simulink model "a"  (R2015a)
settings: Solver=ode3  StartTime=0.0  StopTime=20  FixedStep=2e-5  RelTol=2e-5
libraries: commchan3 x1, dsparch4 x1, commsink2 x1, commutil2 x1, commrandsrc2 x1, dspsigops x1
settings Model: Creator=Win 10  LastModifiedBy=Win 10

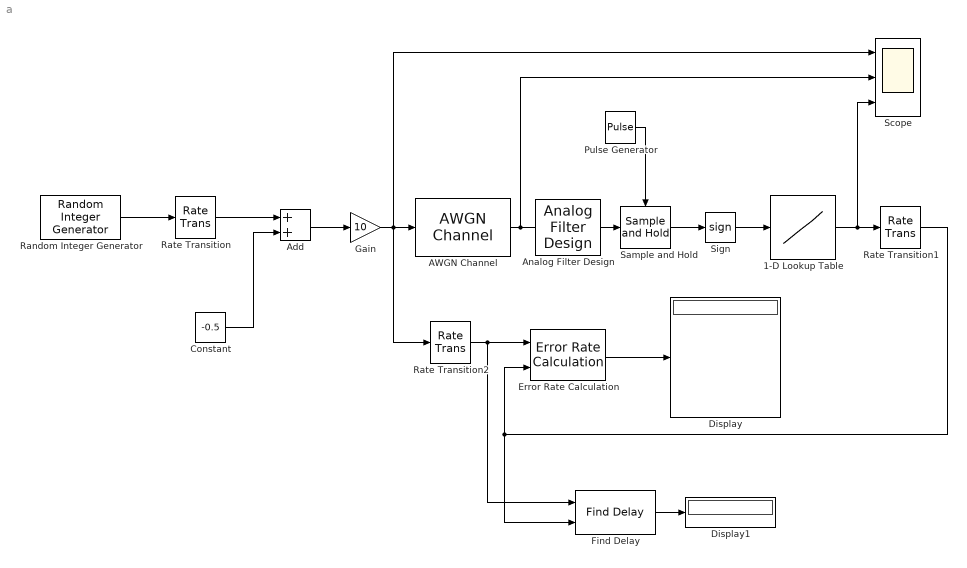
== system a ==
  1-D Lookup Table : Lookup_n-D  NumberOfTableDimensions=1  BreakpointsForDimension1=[-5:5]  Table=tanh([-5:5])  InternalRulePriority=Speed  RndMeth=Simplest  InputSameDT=on
  AWGN Channel : commchan3/AWGN Channel  InputProcessing=Columns as channels (frame based)  seed=67  noiseMode=Variance from mask  EbNodB=10  EsNodB=10  SNRdB=10  bitsPerSym=1  Ps=1  Tsym=1  variance=0
  Add : Sum
  Analog Filter Design : dsparch4/Analog Filter Design  method=Chebyshev I  filttype=Lowpass  N=9  Wlo=1200  Whi=80  Rp=0.1  Rs=40
  Constant : Constant  Value=-0.5
  Display : Display
      settings: Decimation=3
  Display1 : Display
  Error Rate Calculation : commsink2/Error Rate Calculation  N=0  st_delay=0  cp_mode=Entire frame  subframe=[]  PMode=Port  WsName=ErrorVec  RsMode2=off  stop=off  numErr=100  maxBits=1e6
  Find Delay : commutil2/Find Delay  corrLength=200  chgSigOP=off  stopUpdate=off  numConstDelay=3
  Gain : Gain  Gain=10
  Pulse Generator : DiscretePulseGenerator  PulseType=Time based  Period=1/2000  PulseWidth=20
  Random Integer Generator : commrandsrc2/Random Integer Generator  mul=2  seed=37  Ts=1/1000  frameBased=off  sampPerFrame=1  orient=off  outDataType=double
  Rate Transition : RateTransition
  Rate Transition1 : RateTransition  OutPortSampleTime=1/1000
  Rate Transition2 : RateTransition  OutPortSampleTime=1/1000
  Sample and Hold : dspsigops/Sample and Hold  trig=Rising edge  initCond=0  latchinput=off
  Scope : Scope  NumInputPorts=3
      settings: YMin=-5~-5~-5  YMax=5~5~5
  Sign : Signum
  wires:
  Random Integer Generator/1 -> Rate Transition/1
  Rate Transition/1 -> Add/1
  Constant/1 -> Add/2
  Add/1 -> Gain/1
  Gain/1 -> Rate Transition2/1, Scope/1, AWGN Channel/1
  AWGN Channel/1 -> Sample and Hold/1, Scope/2
  Pulse Generator/1 -> Sample and Hold/Trigger
  Sample and Hold/1 -> Sign/1
  1-D Lookup Table/1 -> Scope/3, Rate Transition1/1
  Sign/1 -> 1-D Lookup Table/1
  Rate Transition2/1 -> Find Delay/1, Error Rate Calculation/1
  Error Rate Calculation/1 -> Display/1
  Rate Transition1/1 -> Find Delay/2, Error Rate Calculation/2
  Find Delay/1 -> Display1/1
